simulink model "gm_SECTION10_2"  (R2018b)
settings: Solver=FixedStepDiscrete  StartTime=0.0  StopTime=10.0  RelTol=1e-3
libraries: hdlmdlgenlib x4, simulink x1
settings Model: Creator=ESPINO NOTEBOOK  LastModifiedBy=ESPINO NOTEBOOK
settings DataIOCC: LimitDataPoints=on  SaveOutput=off  SaveTime=off
settings OptimizationCC: BlockReduction=off  ConditionallyExecuteInputs=off  DefaultParameterBehavior=Inlined  LifeSpan=inf
settings DebuggingCC: AlgebraicLoopMsg=error  InheritedTsInSrcMsg=none  SingleTaskRateTransMsg=error  AllowSymbolicDim=off  StrictBusMsg=ErrorOnBusTreatedAsVector  SFUnexpectedBacktrackingDiag=warning  SFNoUnconditionalDefaultTransitionDiag=warning  SFExecutionAtInitializationDiag=none
settings HardwareCC: ProdBitPerPointer=32  ProdBitPerSizeT=32  ProdBitPerPtrDiffT=32  ProdLargestAtomicFloat=None  ProdIntDivRoundTo=Undefined  ProdEndianess=Unspecified  ProdWordSize=32  ProdHWDeviceType=ASIC/FPGA->ASIC/FPGA  ProdEqTarget=off
settings SFSimCC: SimUseLocalCustomCode=off
settings RTWCC: RTWUseLocalCustomCode=off
settings CodeAppCC: StateflowObjectComments=on
settings GRTTargetCC: TargetLangStandard=C89/C90 (ANSI)  GeneratePreprocessorConditionals=Disable all
settings ConfigComp: CovScope=ReferencedModels  CovMetricSettings=dw  CovHtmlReporting=on  CovSaveCumulativeToWorkspaceVar=on  CovSaveSingleToWorkspaceVar=on  CovExternalEMLEnable=off  CovSFcnEnable=off

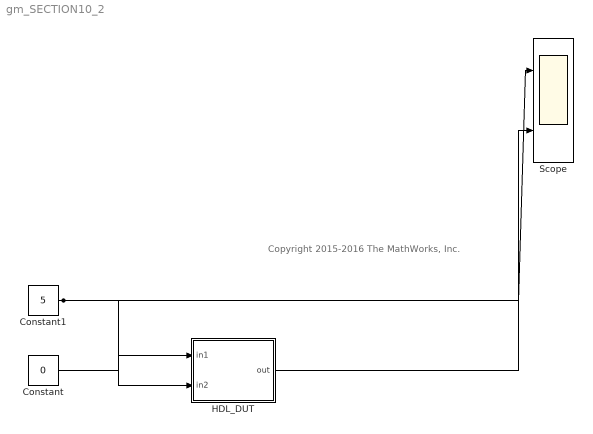
== system gm_SECTION10_2 ==
  note: Copyright 2015-2016 The MathWorks, Inc.
  Constant : Constant  Value=0  OutDataTypeStr=fixdt(0, 4, 0)  SampleTime=-1
  Constant1 : Constant  Value=5  OutDataTypeStr=fixdt(1, 32, 10)  SampleTime=-1
  HDL_DUT : Subsystem
  Scope : Scope  NumInputPorts=2
  wires:
  Constant/1 -> HDL_DUT/1(in1)
  Constant1/1 -> Scope/1, HDL_DUT/2(in2)
  HDL_DUT/1(out) -> Scope/2

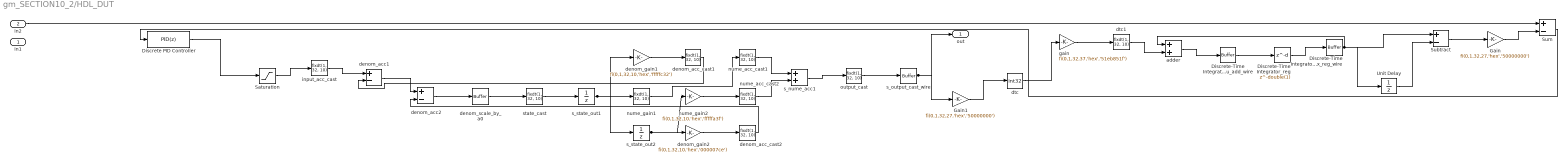
== system gm_SECTION10_2/HDL_DUT ==
  in1 : Inport  OutDataTypeStr=fixdt(0, 4, 0)  PortDimensions=1  SampleTime=0.01
  in2 : Inport  Port=2  OutDataTypeStr=fixdt(1, 32, 10)  PortDimensions=1  SampleTime=0.01
  Discrete PID Controller : simulink/Continuous/PID Controller  Controller=PID  Form=Parallel  TimeDomain=Discrete-time  SampleTime=0.01  IntegratorMethod=Forward Euler  FilterMethod=Forward Euler  ControllerParametersSource=internal  P=0.10  I=0.6426  D=0.00047  UseFilter=on  N=20.74  TunerSelectOption=Transfer Function Based (PID Tuner App)  InitialConditionSource=internal  InitialConditionForIntegrator=0  InitialConditionForFilter=0  DifferentiatorICPrevScaledInput=0  ExternalReset=none  TrackingMode=off  Kt=1  LimitOutput=off  UpperSaturationLimit=inf  LowerSaturationLimit=-inf  LinearizeAsGain=off  AntiWindupMode=none  Kb=1  RndMeth=Round  PGainOutDataTypeStr=fixdt(1,32,10)  PProdOutDataTypeStr=fixdt(1,32,10)  POutMin=[]  POutMax=[]  IGainOutDataTypeStr=fixdt(1,32,10)  IProdOutDataTypeStr=fixdt(1,32,10)  IOutMin=[]  IOutMax=[]  DGainOutDataTypeStr=fixdt(1,32,10)  DProdOutDataTypeStr=fixdt(1,32,10)  DOutMin=[]  DOutMax=[]  NGainOutDataTypeStr=fixdt(1,32,10)  NProdOutDataTypeStr=fixdt(1,32,10)  NOutMin=[]  NOutMax=[]  SumOutDataTypeStr=fixdt(1,32,10)  SumOutMin=[]  SumOutMax=[]  SaturationOutMin=[]  SaturationOutMax=[]  PParamDataTypeStr=fixdt(1,32,10)  PParamMin=[]  PParamMax=[]  IParamDataTypeStr=fixdt(1,32,10)  IParamMin=[]  IParamMax=[]  DParamDataTypeStr=fixdt(1,32,10)  DParamMin=[]  DParamMax=[]  NParamDataTypeStr=fixdt(1,32,10)  NParamMin=[]  NParamMax=[]  KbParamMin=[]  KbParamMax=[]  KtParamMin=[]  KtParamMax=[]  KbOutMin=[]  KbOutMax=[]  KtOutMin=[]  KtOutMax=[]  IntegratorOutDataTypeStr=fixdt(1,32,10)  IntegratorOutMin=[]  IntegratorOutMax=[]  FilterOutDataTypeStr=fixdt(1,32,10)  FilterOutMin=[]  FilterOutMax=[]  SumI1OutMin=[]  SumI1OutMax=[]  SumI2OutMin=[]  SumI2OutMax=[]  SumI3OutMin=[]  SumI3OutMax=[]  SumI4OutMin=[]  SumI4OutMax=[]  SumDOutDataTypeStr=fixdt(1,32,10)  SumDOutMin=[]  SumDOutMax=[]  SumAccumDataTypeStr=fixdt(1,32,10)  SumDAccumDataTypeStr=fixdt(1,32,10)  DifferentiatorOutMin=[]  DifferentiatorOutMax=[]  FilterDiffOutCoefMin=[]  FilterDiffOutCoefMax=[]  ReciprocalOutMin=[]  ReciprocalOutMax=[]  SumDenOutMin=[]  SumDenOutMax=[]  SumNumOutMin=[]  SumNumOutMax=[]  DivideOutMin=[]  DivideOutMax=[]  IntegratorContinuousStateAttributes=''  IntegratorStateMustResolveToSignalObject=off  IntegratorRTWStateStorageClass=Auto  FilterContinuousStateAttributes=''  FilterStateMustResolveToSignalObject=off  FilterRTWStateStorageClass=Auto  ParallelPVariant=InternalParameters  IdealPVariant=Disabled  IVariant=InternalParameters  DVariant=InternalParameters  IntegratorVariant=Discrete  SatVariant=Disabled  AWVariant=Passthrough  PCopyVariant=Disabled  TRVariant=Disabled  FdbkBlocksVariant=Forward  IdealPFdbkVariant=Disabled  SatFdbkVariant=Disabled  DerivativeFilterVariant=ForwardEulerFilter  NVariant=InternalParameters  NCopyVariant=Disabled  FilterICVariant=InternalICsFilter  IntegratorICVariant=InternalICs  ExternalResetVariant=Disabled  TRSumVariant=Passthrough  SumFdbkVariant=Disabled  SumVariant=Sum_PID
  Discrete-Time Integrator_reg : Delay  DelayLength=double(1)  InitialCondition=0  InputProcessing=Inherited  SampleTime=0.01
  Discrete-Time Integrator_u_add_wire : hdlmdlgenlib/Buffer
      settings: SourceProductName=HDL Coder  SourceProductBaseCode=HD
  Discrete-Time Integrator_x_reg_wire : hdlmdlgenlib/Buffer
      settings: SourceProductName=HDL Coder  SourceProductBaseCode=HD
  Gain : Gain  Gain=fi(0,1,32,27,'hex','50000000')  ParamDataTypeStr=fixdt(1, 32, 27)  OutDataTypeStr=fixdt(1, 32, 10)  SampleTime=0.01
  Gain1 : Gain  Gain=fi(0,1,32,27,'hex','50000000')  ParamDataTypeStr=fixdt(1, 32, 27)  OutDataTypeStr=fixdt(1, 32, 10)  SampleTime=0.01
  Saturation : Saturate  UpperLimit=fi(0,1,32,10,'hex','00019000')  LowerLimit=fi(0,1,32,10,'hex','00000000')  SampleTime=0.01  OutDataTypeStr=fixdt(1, 32, 10)
  Subtract : Sum  Inputs=+-  AccumDataTypeStr=fixdt(1, 33, 10)  OutDataTypeStr=fixdt(1, 32, 10)  SampleTime=0.01
  Sum : Sum  Inputs=+-  AccumDataTypeStr=fixdt(1, 32, 10)  OutDataTypeStr=fixdt(1, 32, 10)  SampleTime=0.01
  Unit Delay : UnitDelay  InitialCondition=fi(0,1,32,10,'hex','00000000')  SampleTime=0.01
  adder : Sum  AccumDataTypeStr=fixdt(1, 32, 10)  OutDataTypeStr=fixdt(1, 32, 10)  SampleTime=0.01
  denom_acc1 : Sum  Inputs=+-  AccumDataTypeStr=fixdt(1, 32, 10)  OutDataTypeStr=fixdt(1, 32, 10)  SampleTime=0.01
  denom_acc2 : Sum  Inputs=+-  AccumDataTypeStr=fixdt(1, 32, 10)  OutDataTypeStr=fixdt(1, 32, 10)  SampleTime=0.01
  denom_acc_cast1 : DataTypeConversion  OutDataTypeStr=fixdt(1, 32, 10)  SampleTime=0.01
  denom_acc_cast2 : DataTypeConversion  OutDataTypeStr=fixdt(1, 32, 10)  SampleTime=0.01
  denom_gain1 : Gain  Gain=fi(0,1,32,10,'hex','fffffc32')  ParamDataTypeStr=fixdt(1, 32, 10)  OutDataTypeStr=fixdt(1, 32, 10)  SampleTime=0.01
  denom_gain2 : Gain  Gain=fi(0,1,32,10,'hex','000007ce')  ParamDataTypeStr=fixdt(1, 32, 10)  OutDataTypeStr=fixdt(1, 32, 10)  SampleTime=0.01
  denom_scale_by_a0 : hdlmdlgenlib/Buffer
      settings: SourceProductName=HDL Coder  SourceProductBaseCode=HD
  dtc : DataTypeConversion  OutDataTypeStr=int32  ConvertRealWorld=Stored Integer (SI)  SampleTime=0.01
  dtc1 : DataTypeConversion  OutDataTypeStr=fixdt(1, 32, 10)  ConvertRealWorld=Stored Integer (SI)  SampleTime=0.01
  gain : Gain  Gain=fi(0,1,32,37,'hex','51eb851f')  ParamDataTypeStr=fixdt(1, 32, 37)  OutDataTypeStr=int32  SampleTime=0.01
  input_acc_cast : DataTypeConversion  OutDataTypeStr=fixdt(1, 32, 10)  SampleTime=0.01
  nume_acc_cast1 : DataTypeConversion  OutDataTypeStr=fixdt(1, 32, 10)  SampleTime=0.01
  nume_acc_cast2 : DataTypeConversion  OutDataTypeStr=fixdt(1, 32, 10)  SampleTime=0.01
  nume_gain1 : DataTypeConversion  OutDataTypeStr=fixdt(1, 32, 10)  SampleTime=0.01
  nume_gain2 : Gain  Gain=fi(0,1,32,10,'hex','fffffa3f')  ParamDataTypeStr=fixdt(1, 32, 10)  OutDataTypeStr=fixdt(1, 32, 10)  SampleTime=0.01
  output_cast : DataTypeConversion  OutDataTypeStr=fixdt(1, 32, 10)  SampleTime=0.01
  s_nume_acc1 : Sum  OutDataTypeStr=fixdt(1, 32, 10)  SampleTime=0.01
  s_output_cast_wire : hdlmdlgenlib/Buffer
      settings: SourceProductName=HDL Coder  SourceProductBaseCode=HD
  s_state_out1 : UnitDelay  InitialCondition=fi(0,1,32,10,'hex','00000000')  SampleTime=0.01
  s_state_out2 : UnitDelay  InitialCondition=fi(0,1,32,10,'hex','00000000')  SampleTime=0.01
  state_cast : DataTypeConversion  OutDataTypeStr=fixdt(1, 32, 10)  SampleTime=0.01
  out : Outport
  wires:
  in2/1 -> Sum/1
  s_output_cast_wire/1 -> Gain1/1, out/1
  Discrete PID Controller/1 -> Saturation/1
  Discrete-Time Integrator_x_reg_wire/1 -> Subtract/1, Unit Delay/1, adder/1
  Gain/1 -> Sum/2
  Gain1/1 -> dtc/1
  Saturation/1 -> input_acc_cast/1
  Subtract/1 -> Gain/1
  Sum/1 -> Discrete PID Controller/1
  Unit Delay/1 -> Subtract/2
  input_acc_cast/1 -> denom_acc1/1
  denom_acc_cast1/1 -> denom_acc1/2
  denom_acc1/1 -> denom_acc2/1
  denom_acc_cast2/1 -> denom_acc2/2
  denom_acc2/1 -> denom_scale_by_a0/1
  denom_scale_by_a0/1 -> state_cast/1
  state_cast/1 -> s_state_out1/1
  s_state_out1/1 -> nume_gain1/1, denom_gain1/1, s_state_out2/1
  s_state_out2/1 -> nume_gain2/1, denom_gain2/1
  denom_gain1/1 -> denom_acc_cast1/1
  denom_gain2/1 -> denom_acc_cast2/1
  nume_gain1/1 -> nume_acc_cast1/1
  nume_acc_cast1/1 -> s_nume_acc1/1
  nume_gain2/1 -> nume_acc_cast2/1
  nume_acc_cast2/1 -> s_nume_acc1/2
  s_nume_acc1/1 -> output_cast/1
  output_cast/1 -> s_output_cast_wire/1
  dtc/1 -> gain/1
  gain/1 -> dtc1/1
  dtc1/1 -> adder/2
  adder/1 -> Discrete-Time Integrator_u_add_wire/1
  Discrete-Time Integrator_u_add_wire/1 -> Discrete-Time Integrator_reg/1
  Discrete-Time Integrator_reg/1 -> Discrete-Time Integrator_x_reg_wire/1
